simulink model "Smart_City_QCar2_VIRTUAL_car5"  (R2024b)
settings: Solver=ode1  StartTime=0.0  StopTime=inf  FixedStep=Controller_Sample_Time  RelTol=1e-3  EnableMultiTasking=on
values from neighbouring files (symbols this model uses):
  Audio_Sample_Time = 0.3    [Setup_QCar1and2_params.m]
  cameraStepSize = 3e-2    (= 0.03)    [Setup_QCar1and2_params.m]
  CSI_Sample_Time = 1/60    (= 0.0166666666667)    [Setup_QCar1and2_params.m]
  ImageDisplay_Sample_Time = CSI_Sample_Time*6    (= 0.1)    [Setup_QCar1and2_params.m]
  Initialization_Time = 5    [Setup_QCar1and2_params.m]
  LiDAR_Sample_Time = CSI_Sample_Time*3    (= 0.05)    [Setup_QCar1and2_params.m]
  map_mask = [1 1 1 0 0 1 0]    [Setup_QCar1and2_params.m]
  NN_Sample_Time = RealSense_Sample_Time*1    (= 0.0333333333333)    [Setup_QCar1and2_params.m]
  path_x = [0.826 0.836 0.846 0.856 0.866 0.876 0.886 0.896 0.906 0.916 0.926 0.936 ... (740 elements, 740x1)]    [SDCS_Paths_7.mat]
  path_x2 = [-0.614 -0.604 -0.594 -0.584 -0.574 -0.564 -0.554 -0.544 -0.534 -0.524 -0.514 -0.504 ... (1090 elements, 1090x1)]    [SDCS_Paths_7.mat]
  path_x3 = [-0.614 -0.603821428571 -0.593642857143 -0.583464285714 -0.573285714286 -0.563107142857 -0.552928571429 -0.54275 -0.532571428571 -0.522392857143 -0.512214285714 -0.502035714286 ... (714 elements, 714x1)]    [SDCS_Paths_7.mat]
  path_x4 = [-0.614 -0.604 -0.594 -0.584 -0.574 -0.564 -0.554 -0.544 -0.534 -0.524 -0.514 -0.504 ... (1761 elements, 1761x1)]    [SDCS_Paths_7.mat]
  path_x5 = [1.436 1.42588571429 1.41577142857 1.40565714286 1.39554285714 1.38542857143 1.37531428571 1.3652 1.35508571429 1.34497142857 1.33485714286 1.32474285714 ... (574 elements, 574x1)]    [SDCS_Paths_7.mat]
  path_x6 = [1.436 1.42588571429 1.41577142857 1.40565714286 1.39554285714 1.38542857143 1.37531428571 1.3652 1.35508571429 1.34497142857 1.33485714286 1.32474285714 ... (1288 elements, 1288x1)]    [SDCS_Paths_7.mat]
  path_x7 = [-1.5778487585 -1.56959877056 -1.56127865467 -1.55288878259 -1.54442952915 -1.53590127231 -1.52730439309 -1.51863927561 -1.50990630701 -1.50110587746 -1.49223838016 -1.4833042113 ... (2260 elements, 2260x1)]    [SDCS_Paths_7.mat]
  path_y = [-1.0887 -1.0887 -1.0887 -1.0887 -1.0887 -1.0887 -1.0887 -1.0887 -1.0887 -1.0887 -1.0887 -1.0887 ... (740 elements, 740x1)]    [SDCS_Paths_7.mat]
  path_y2 = [-1.0887 -1.0887 -1.0887 -1.0887 -1.0887 -1.0887 -1.0887 -1.0887 -1.0887 -1.0887 -1.0887 -1.0887 ... (1090 elements, 1090x1)]    [SDCS_Paths_7.mat]
  path_y3 = [-1.0887 -1.0887 -1.0887 -1.0887 -1.0887 -1.0887 -1.0887 -1.0887 -1.0887 -1.0887 -1.0887 -1.0887 ... (714 elements, 714x1)]    [SDCS_Paths_7.mat]
  path_y4 = [-1.0887 -1.0887 -1.0887 -1.0887 -1.0887 -1.0887 -1.0887 -1.0887 -1.0887 -1.0887 -1.0887 -1.0887 ... (1761 elements, 1761x1)]    [SDCS_Paths_7.mat]
  path_y5 = [-0.8157 -0.8157 -0.8157 -0.8157 -0.8157 -0.8157 -0.8157 -0.8157 -0.8157 -0.8157 -0.8157 -0.8157 ... (574 elements, 574x1)]    [SDCS_Paths_7.mat]
  path_y6 = [-0.8157 -0.8157 -0.8157 -0.8157 -0.8157 -0.8157 -0.8157 -0.8157 -0.8157 -0.8157 -0.8157 -0.8157 ... (1288 elements, 1288x1)]    [SDCS_Paths_7.mat]
  path_y7 = [-0.614490295955 -0.61974988896 -0.624981792226 -0.630185771997 -0.635361595765 -0.640509032279 -0.645627851559 -0.6507178249 -0.655778724888 -0.660810325409 -0.665812401655 -0.670784730139 ... (2260 elements, 2260x1)]    [SDCS_Paths_7.mat]
  RealSense_Sample_Time = CSI_Sample_Time*2    (= 0.0333333333333)    [Setup_QCar1and2_params.m]
undefined symbols (not defined in the file or in its folder): DiscIntNeverNeededParam, gcbh, Joystick_Sample_Time, JPEG, qc_get_step_size, video_display_show
libraries: quarc_library x61, simulink_extras x9, simulink x5
(part 4 of 4)

== matlab function Smart_City_QCar2_VIRTUAL_car5/Speed & Steering Commander/Path Commander/Path 5  Look Ahead Generator/Windowed Closest Point Locator *Feedback the location1 ==
  data: x input; location output; y input; x_array input; y_array input; window input; global_search input; distance output; previous_location input
function [location,distance] = find_closest_window_point(x,y,x_array,y_array, window, global_search, previous_location)
distance = 1e6;
location = previous_location;
array_length = length (x_array);

if (global_search == 1)
    
    %Search the whole array (usually at startup)
    for i =1:array_length
        d = (x-x_array(i))^2 + (y-y_array(i))^2;
        if d < distance
            distance = d;
            location = i;
        end
    end
    
else
    
    if (location + window) > array_length
        %We need to wrap from the end
        % loop one - end of array:
        for i = (location-window):array_length
            d = (x-x_array(i))^2 + (y-y_array(i))^2;
            if d < distance
                distance = d;
                location = i;
            end
        end
        % loop two - start of array:
        for i = 1:(location+window-array_length)
            d = (x-x_array(i))^2 + (y-y_array(i))^2;
            if d < distance
                distance = d;
                location = i;
            end
        end
        
    elseif (location-window) < 1
        %We need to wrap from the beginning
        % loop one - end of array:
        for i = (array_length+location-window):array_length
            d = (x-x_array(i))^2 + (y-y_array(i))^2;
            if d < distance
                distance = d;
                location = i;
            end
        end
        % loop two - start of array:
        for i = 1:(location+window)
            d = (x-x_array(i))^2 + (y-y_array(i))^2;
            if d < distance
                distance = d;
                location = i;
            end
        end
        
    else
        %no need to wrap
        for i = (location-window):(location+window)
            d = (x-x_array(i))^2 + (y-y_array(i))^2;
            if d < distance
                distance = d;
                location = i;
            end
        end
    end
    
end
distance = sqrt(distance);
end

== matlab function Smart_City_QCar2_VIRTUAL_car5/Speed & Steering Commander/Path Commander/Path 6  Look Ahead Generator/Windowed Closest Point Locator *Feedback the location1 ==
  data: x input; location output; y input; x_array input; y_array input; window input; global_search input; distance output; previous_location input
function [location,distance] = find_closest_window_point(x,y,x_array,y_array, window, global_search, previous_location)
distance = 1e6;
location = previous_location;
array_length = length (x_array);

if (global_search == 1)
    
    %Search the whole array (usually at startup)
    for i =1:array_length
        d = (x-x_array(i))^2 + (y-y_array(i))^2;
        if d < distance
            distance = d;
            location = i;
        end
    end
    
else
    
    if (location + window) > array_length
        %We need to wrap from the end
        % loop one - end of array:
        for i = (location-window):array_length
            d = (x-x_array(i))^2 + (y-y_array(i))^2;
            if d < distance
                distance = d;
                location = i;
            end
        end
        % loop two - start of array:
        for i = 1:(location+window-array_length)
            d = (x-x_array(i))^2 + (y-y_array(i))^2;
            if d < distance
                distance = d;
                location = i;
            end
        end
        
    elseif (location-window) < 1
        %We need to wrap from the beginning
        % loop one - end of array:
        for i = (array_length+location-window):array_length
            d = (x-x_array(i))^2 + (y-y_array(i))^2;
            if d < distance
                distance = d;
                location = i;
            end
        end
        % loop two - start of array:
        for i = 1:(location+window)
            d = (x-x_array(i))^2 + (y-y_array(i))^2;
            if d < distance
                distance = d;
                location = i;
            end
        end
        
    else
        %no need to wrap
        for i = (location-window):(location+window)
            d = (x-x_array(i))^2 + (y-y_array(i))^2;
            if d < distance
                distance = d;
                location = i;
            end
        end
    end
    
end
distance = sqrt(distance);
end

== matlab function Smart_City_QCar2_VIRTUAL_car5/Infrastructure/Find Closest Car/MATLAB Function ==
  data: x_car input; distance output; y_car input; x_vector input; y_vector input; car_index input; heading input; proximity_radius input; proximity_scan_window input; max_distance input; distance_vector output; heading_vector output
function [distance, distance_vector, heading_vector] = proximity_sensor (x_car, y_car, x_vector, y_vector, car_index, heading, proximity_radius, proximity_scan_window, max_distance)
distance = max_distance;
distance_vector = max_distance + 0*x_vector;
heading_vector = 2*pi +  0*x_vector;

for i = 1:length (x_vector)
    if (i ~= car_index)
        distance_vector(i) = sqrt ((x_car - x_vector(i))^2 + (y_car - y_vector(i))^2);
        heading_vector(i) = atan2( (y_vector(i) - y_car), (x_vector(i) - x_car)) - heading;
        if (heading_vector(i) > pi)
            heading_vector(i) = heading_vector(i) - 2*pi;
        elseif (heading_vector(i) < -pi)
            heading_vector(i) = heading_vector(i) + 2*pi;
        end
        if ((distance_vector(i) < distance) && (abs (heading_vector(i)) <= proximity_scan_window))
            distance =  distance_vector(i);
        end
       
    end
end

== matlab function Smart_City_QCar2_VIRTUAL_car5/Infrastructure/Find Closest Car/MATLAB Function1 ==
  data: speed input; proximity_scan_window output; max_speed input; min_window input; max_window input
function proximity_scan_window = scan_window_generator(speed, max_speed, min_window, max_window)
%#codegen
proximity_scan_window = min_window + speed*(max_window - min_window) / max_speed;
end

== matlab function Smart_City_QCar2_VIRTUAL_car5/Speed & Steering Commander/Traffic Zone 1/MATLAB Function2 ==
  data: Previous_State input; Speed_In input; Speed_Multi input; In_Zone input; Traffic_State output; Speed_Out output; Traffic_Light input
function [Traffic_State, Speed_Out]  = Traffic_Controller (Previous_State, Speed_In, Speed_Multi, In_Zone, Traffic_Light)
%#codegen
Traffic_State = Previous_State;
Speed_Out = Speed_In;

switch Traffic_State
    % Case 1 - Normal - either not in zone or green light, Case 2 - red
    % light and in zone
    
    case 1
        % Green light or not in zone
        Speed_Out = Speed_In;
        if (Traffic_Light == 0) && (In_Zone == 1)
            % Caught in the traffic controller's web!
            Traffic_State = 2;
        end
        
    case 2
        % Red light state
        Speed_Out = Speed_In * Speed_Multi;
        
        if (Traffic_Light == 1)
            % Green Light
            Traffic_State = 1;
        end
        
end
end

== matlab function Smart_City_QCar2_VIRTUAL_car5/RealSense Camera/obstacleDetection Markham March 22/Steering based image subselector ==
  data: pts output; depth input; distance output; steering input; minDistance input; maxDistance input; width input; height input; vertCenter input; maxSteering input; reduction input; maxSteeringWidth input; median_pts output; mean_pts output; min_pts output; max_pts output; num_pts output; pt_25 output; mean_middle output
function [pts, distance, median_pts, mean_pts, min_pts, max_pts, num_pts, pt_25, mean_middle] = estimateDepthInRegion(depth, steering, minDistance, maxDistance, width, height, vertCenter, maxSteering, reduction, maxSteeringWidth)
% Input: 640 x 480
[ROW, COL] = size(depth);
mark = COL/2 - (steering*(COL/2 - width/2)/maxSteering);
applied_width = max(width - abs(steering/maxSteeringWidth)*reduction*width, 60);
left_w = max(mark+1-(applied_width/2), 0); % pick the left end, but never let it get negative
right_w = min(left_w + applied_width, COL); % pick the right end, but never past the image width
upper_h = max(ROW*vertCenter-height/2+1, 0); % pick the upper end, but never let it get negative
lower_h = min(ROW*vertCenter+height/2, ROW); % pick the lower end, but never let it go past the image height
depth(:,1:40) = maxDistance; %this is to remove artifacts in the camera's left section
region = double(depth(upper_h:lower_h, left_w:right_w)); 
pts = [upper_h, left_w; upper_h, right_w; lower_h, right_w; lower_h, left_w; upper_h, left_w];

% reshape region of interest into 1D array
u_flat = reshape(region, 1, []);
% store a temp comparison matrix the size of u_flat
temp = maxDistance*ones(1, length(u_flat));

% compare u_flat to min and max distance
for i = 1:length(u_flat)
    % if u_flat is between min and max distance, store in temp array
    if (u_flat(i) >= minDistance) && (u_flat(i) <= maxDistance)
        temp(i) = u_flat(i);
    end
end

% u_flat(u_flat < minDistance) = [];
% u_flat(u_flat > maxDistance) = [];
% distance = mean(mean(u_flat));
distance = min(temp(:));
num_pts = 0;
median_pts = 0;
min_pts = 0;
mean_pts = 0;
max_pts = 0;

num_pts = length(temp);
median_pts = median (temp);
min_pts = min (temp);
max_pts = max (temp);
mean_pts = mean (temp);

% sort temp array small to large
sorted_points = sort (temp);
% pt_25 = 25% smallest distance in the array
pt_25 = sorted_points (floor(num_pts/4));
smaller_points = sorted_points (floor(num_pts/4):floor(num_pts*3/4));
mean_middle = mean (smaller_points);

== matlab function Smart_City_QCar2_VIRTUAL_car5/Randomizer1/MATLAB Function ==
  data: Previous_Path input; Previous_Speed input; Path_Options input; Speed_Cmd_Base input; randomize input; Desired_Path output; Desired_Speed output; Accel_Limit output
function [Desired_Path, Desired_Speed,  Accel_Limit] = Random_Driving(Previous_Path, Previous_Speed, Path_Options, Speed_Cmd_Base, randomize)

% Define Params
Desired_Path = Previous_Path;
Desired_Speed = Previous_Speed;
Accel_Limit = 0;
num_Path_Options = sum (Path_Options);

% if it is time to switch paths and there are viable options
if (randomize == 1) && (num_Path_Options > 0)
    random_Path = randi (num_Path_Options);
    valid_Paths = find (Path_Options);
    Desired_Path = valid_Paths (random_Path);
    Desired_Speed = Speed_Cmd_Base*randi(2);
    Accel_Limit = 0.1*randi(2);
end

% if the desired path is not an option maintain current path
if (Path_Options (Desired_Path) == 0)
    Desired_Path = Previous_Path;
end
end

== matlab function Smart_City_QCar2_VIRTUAL_car5/Speed & Steering Commander/Path Commander/Path 3  Look Ahead Generator/Windowed Closest Point Locator *Feedback the location1 ==
  data: x input; location output; y input; x_array input; y_array input; window input; global_search input; distance output; previous_location input
function [location,distance] = find_closest_window_point(x,y,x_array,y_array, window, global_search, previous_location)
distance = 1e6;
location = previous_location;
array_length = length (x_array);

if (global_search == 1)
    
    %Search the whole array (usually at startup)
    for i =1:array_length
        d = (x-x_array(i))^2 + (y-y_array(i))^2;
        if d < distance
            distance = d;
            location = i;
        end
    end
    
else
    
    if (location + window) > array_length
        %We need to wrap from the end
        % loop one - end of array:
        for i = (location-window):array_length
            d = (x-x_array(i))^2 + (y-y_array(i))^2;
            if d < distance
                distance = d;
                location = i;
            end
        end
        % loop two - start of array:
        for i = 1:(location+window-array_length)
            d = (x-x_array(i))^2 + (y-y_array(i))^2;
            if d < distance
                distance = d;
                location = i;
            end
        end
        
    elseif (location-window) < 1
        %We need to wrap from the beginning
        % loop one - end of array:
        for i = (array_length+location-window):array_length
            d = (x-x_array(i))^2 + (y-y_array(i))^2;
            if d < distance
                distance = d;
                location = i;
            end
        end
        % loop two - start of array:
        for i = 1:(location+window)
            d = (x-x_array(i))^2 + (y-y_array(i))^2;
            if d < distance
                distance = d;
                location = i;
            end
        end
        
    else
        %no need to wrap
        for i = (location-window):(location+window)
            d = (x-x_array(i))^2 + (y-y_array(i))^2;
            if d < distance
                distance = d;
                location = i;
            end
        end
    end
    
end
distance = sqrt(distance);
end

== matlab function Smart_City_QCar2_VIRTUAL_car5/QCar/To//From Simulation/Transmit Fcn ==
  settings: updateMethod=DISCRETE  sampleTime=qc_get_step_size
  data: Packet output size=65537; ServerState input; SendUpdate input; Enable output; DeviceNumber input; Forward_And_Steering input; Lights input; EnableCameras input; LEDStrip input; LEDStripNew input; EnableLIDAR input
function [Packet,Enable] = QCar2ApplicationWorkspaceMakePacketData(ServerState, SendUpdate, DeviceNumber, Forward_And_Steering, Lights, EnableCameras, LEDStrip, LEDStripNew, EnableLIDAR) 

% Be sure to set the maximum signal size of the variable size Packet port 
% in Simulink->Edit Data of the editor window.  Size should be 65537 or
% larger to ensure that the stream server generates a 4 byte packet size.

%% Setup
persistent LastServerState;
persistent LastLEDStrip;

if isempty(LastServerState)
    LastServerState = uint8(0);

    % Initialize with -1 to ensure it will always send the first update.
    LastLEDStrip = -1*ones(3,33);
end

Enable = 0;
Packet = uint8([]);


%% Send new State Container or On connection
% Previous state processed, send a new one
if (SendUpdate) || ((ServerState == 2) && (LastServerState ~= 2))
    Packet = QCar2MakeCommandVelocityStateContainer(DeviceNumber, Forward_And_Steering, Lights);
    
    for (index = 1:6)
        if (EnableCameras(index))
            Packet = [Packet; QCar2MakeCameraRequestContainer(DeviceNumber, index-1)];
        end
    end

    if (LEDStripNew)
        % This is an expensive operation so only send this if it has
        % changed.
        if ~all(all(LastLEDStrip == LEDStrip))
            LastLEDStrip = LEDStrip;
            Brightness = 10;
            Packet = [Packet; QCar2MakeSetLEDStripContainer(DeviceNumber, LEDStrip, Brightness)];
        end
    end

    if (EnableLIDAR)
        Packet = [Packet; QCar2MakeLidarRequestContainer(DeviceNumber)];
    end
end

%% Transmit
% If we have data to send, enable the transmit
PacketLength = length(Packet);

if (PacketLength > 0)
    % Add magic byte.  This is just for error handling and isn't typically
    % required in simulink, but useful in lower-level languages like Python
    Packet = [uint8(123); Packet];
    
    Enable = 1; 
end


LastServerState = ServerState;
